simulink model "pmsm_ctrl"  (R2018a)
settings: Solver=FixedStepDiscrete  StartTime=0.0  StopTime=3  FixedStep=FastTsample / 10.  RelTol=1e-3  EnableMultiTasking=on
model workspace (MATLAB code in the model file):
  | cmdLim = Simulink.Parameter;
  | cmdLim.Value = 15;
  | cmdLim.Description = 'Limit for controlling the maximum surface command angle.';
  | cmdLim.Min = 0;
  | cmdLim.Max = 90;
  | cmdLim.DocUnits = 'deg';
  | 
  | dispGain = Simulink.Parameter;
  | dispGain.Value = 0.75;
  | dispGain.Description = 'Gain applied to the displacement error.';
  | dispGain.Min = 0;
  | dispGain.Max = [];
  | dispGain.DocUnits = 'deg/sec/deg';
  | 
  | dispLim = Simulink.Parameter;
  | dispLim.Value = 30;
  | dispLim.Description = 'Limit for controlling the maximum commanded angle.';
  | dispLim.Min = 0;
  | dispLim.Max = 180;
  | dispLim.DocUnits = 'deg';
  | 
  | intGain = Simulink.Parameter;
  | intGain.Value = 0.5;
  | intGain.Description = 'Gain applied to the integral error.';
  | intGain.Min = 0;
  | intGain.Max = [];
  | intGain.DocUnits = 'deg/sec/deg/sec';
  | 
  | intLim = Simulink.Parameter;
  | intLim.Value = 5;
  | intLim.Description = 'Limit for controlling the maximum commanded angle.';
  | intLim.Min = 0;
  | intLim.Max = 90;
  | intLim.DocUnits = 'deg';
  | 
  | rateGain = Simulink.Parameter;
  | rateGain.Value = 2;
  | rateGain.Description = 'Gain applied to the rate error.';
  | rateGain.Min = 0;
  | rateGain.Max = [];
  | rateGain.DocUnits = 'deg/deg/sec';
  | 
  | rateLim = Simulink.Parameter;
  | rateLim.Value = 6;
  | rateLim.Description = 'Limit for controlling the maximum commanded angle.';
  | rateLim.Min = 0;
  | rateLim.Max = 180;
  | rateLim.DocUnits = 'deg/sec';
  | 
  | hdgGain = Simulink.Parameter;
  | hdgGain.Value = 0.015;
undefined symbols (not defined in the file): CalMgrSt_T, Cfg_AnglOfsCalPwmDuty, Cfg_AutoCalEnbl, Cfg_EnblDynComp, Cfg_EnblTrajPlan, Cfg_EncCnts, Cfg_EncOfsCalPwmDuty, Cfg_IfbkCtrlBW, Cfg_IndCalPwmDuty, Cfg_Ls, Cfg_MFlux, Cfg_MtrJm, Cfg_MtrKf, Cfg_MtrKtrq, Cfg_PolePairs, Cfg_ResCalPwmDuty, Cfg_Rs, Cfg_SpdCtrlBW, Cfg_SpdSnsEnbl, Cfg_StepToEncCnts, Cfg_UseObsPosEst, Cfg_VBus, DiscIntNeverNeededParam, DistObs_J, EncCntsToRads, MtrCtrlCal_T, MtrCtrlMd, MtrCtrlMd_T, MtrParams, TsFast, TsMain
libraries: ctrl_lib x13, simulink x10, adrc_lib x2, peTransforms x1
(part 2 of 2)

== system pmsm_ctrl/CtrlFast/Field_Oriented_Controller/ifbk_trq_ctrl/IfbkCtrl/ifbk_q_ctrl ==
  IfbkTgt : Inport
  IfbkAct : Inport  Port=2
  Params : Inport  Port=3
  Bus Selector : BusSelector  OutputSignals=Lest,Rest
  Constant : Constant  Value=Cfg_Ls * Cfg_IfbkCtrlBW
  Constant1 : Constant  Value=Cfg_Rs * Cfg_IfbkCtrlBW
  Constant2 : Constant  Value=Cfg_AutoCalEnbl
  Constant3 : Constant  Value=Cfg_IfbkCtrlBW
  Demux : Demux  Outputs=2
  Mux : Mux  Inputs=2
  Mux1 : Mux  Inputs=2
  PI-Ctrl-Varying-Gains : ctrl_lib/PI-Ctrl-Varying-Gains  ts=TsFast  max_lim=12  min_lim=-12
  Product : Product
  Switch : Switch  Criteria=u2 ~= 0
  Ctrl : Outport
  wires:
  IfbkTgt/1 -> PI-Ctrl-Varying-Gains/1
  IfbkAct/1 -> PI-Ctrl-Varying-Gains/2
  Params/1 -> Bus Selector/1
  Bus Selector/2 -> Mux/2  "<Rest>"
  Bus Selector/1 -> Mux/1  "<Lest>"
  Demux/1 -> PI-Ctrl-Varying-Gains/3
  Demux/2 -> PI-Ctrl-Varying-Gains/4
  Constant/1 -> Mux1/1
  Constant1/1 -> Mux1/2
  Switch/1 -> Demux/1
  Mux/1 -> Product/2
  Constant2/1 -> Switch/2
  Mux1/1 -> Switch/3
  Product/1 -> Switch/1
  Constant3/1 -> Product/1
  PI-Ctrl-Varying-Gains/1 -> Ctrl/1

== system pmsm_ctrl/CtrlFast/Field_Oriented_Controller/ifbk_trq_ctrl/IfbkCtrl/mtr_coupling_bemf_comp ==
  ifbk_q_act : Inport
  mtr_spd_act : Inport  Port=2
  ifbk_d_act : Inport  Port=3
  Enable : EnablePort  StatesWhenEnabling=reset
  Add1 : Sum
  Gain : Gain  Gain=-Cfg_Ls  ParamDataTypeStr=single
      settings: AttributesFormatString=%<Gain>
  Gain2 : Gain  Gain=Cfg_MFlux / Cfg_Ls
      settings: AttributesFormatString=%<Gain>
  Gain3 : Gain  Gain=Cfg_Ls
      settings: AttributesFormatString=%<Gain>
  Gain4 : Gain  Gain=Cfg_PolePairs
      settings: AttributesFormatString=%<Gain>
  Product : Product
  Product1 : Product
  ifbk_q_comp : Outport
  ifbk_d_comp : Outport  Port=2
  wires:
  Gain2/1 -> Add1/2
  Product1/1 -> Add1/1
  ifbk_d_act/1 -> Product1/1
  Product/1 -> Gain/1
  Add1/1 -> Gain3/1
  mtr_spd_act/1 -> Gain4/1
  ifbk_q_act/1 -> Product/2
  Gain3/1 -> ifbk_q_comp/1
  Gain/1 -> ifbk_d_comp/1
  Gain4/1 -> Product/1, Product1/2, Gain2/1

== stateflow chart pmsm_ctrl/CalibRoutines/mtr_ind_ident/IndIdCal ==
  state res_id_init
    en, du:
    CtrlMdRqst = MtrCtrlMd_T.CTRL_MD_RAW_PWM;
    PwmRqst = Cfg_IndCalPwmDuty;
    CalMgrStRqst = CalMgrSt_T.ST_IND_ID;
    CalData_L = -1.0;
  state ind_id_actv
    en:
    ifbk_pos = 0;
    ifbk_neg = 0;
    state pos_cycle
      en, du:
      PwmRqst = Cfg_IndCalPwmDuty;
      ifbk_neg += MtrIfbk;
    state neg_cycle
      en, du:
      PwmRqst = -Cfg_IndCalPwmDuty;
      ifbk_pos += MtrIfbk;
    (default) -> pos_cycle
    pos_cycle -> neg_cycle
    neg_cycle -> pos_cycle
  state done
    en, du:
    CtrlMdRqst = MtrCtrlMd_T.CTRL_MD_OFF;
    CalMgrStRqst = CalMgrSt_T.ST_DONE;
    PwmRqst = 0.;
    di_dt = ((ifbk_pos - ifbk_neg) / (TICK_L_CAL / 2.)) / TsMain;
    CalData_L = Cfg_IndCalPwmDuty * (Cfg_VBus/ 2.) / di_dt;
  (default) -> res_id_init
  res_id_init -> ind_id_actv : [after(TICK_L_CAL_WAIT_SETTLE, tick)] // Wait for current / motor to settle.
  ind_id_actv -> done : [after(TICK_L_CAL, tick)]
  data: CtrlMdRqst output; CalMgrStRqst output; PwmRqst output single; MtrIfbk input; CalData_L data_store_memory; MtrParams parameter; Cfg_IndCalPwmDuty parameter single; TICK_L_CAL_WAIT_SETTLE constant uint32 =30; TICK_L_CAL constant uint32 =1000; ifbk_neg local single =0; ifbk_pos local single =0.; di_dt local single =0.; TsMain parameter; Cfg_VBus parameter single

== stateflow chart pmsm_ctrl/CalibRoutines/mtr_ifbk_ofs_ident/ResIdCal ==
  state mtr_angl_ofs_cal_actv
    en, du:
    CtrlMdRqst = MtrCtrlMd_T.CTRL_MD_RAW_PWM;
    PwmRqst = 0.0;
    CalMgrStRqst = CalMgrSt_T.ST_IFBK_OFS_CAL;
    ifbk_abc_sum = get_mtr_ifbk_sum(MtrIfbk);
    CalData_IfbkOfs_Abc[0] = 0.;
    CalData_IfbkOfs_Abc[1] = 0.;
    CalData_IfbkOfs_Abc[2] = 0.;
  state mtr_ifbk_sum_abc = get_mtr_ifbk_sum(mtr_ifbk_abc) [function]
  state mtr_ifbk_avg_abc = get_mtr_ifbk_avg(mtr_ifbk_sum_abc, ncycles) [function]
  state mtr_angl_ofs_cal_done
    en, du:
    CtrlMdRqst = MtrCtrlMd_T.CTRL_MD_OFF;
    CalMgrStRqst = CalMgrSt_T.ST_DONE;
    PwmRqst = 0.0;
    CalData_IfbkOfs_Abc = get_mtr_ifbk_avg(ifbk_abc_sum, TICK_IFBK_OFS_WAIT_SETTLE);
  (default) -> mtr_angl_ofs_cal_actv
  mtr_angl_ofs_cal_actv -> mtr_angl_ofs_cal_done : [after(TICK_IFBK_OFS_WAIT_SETTLE, tick)] // Wait for motor to settle.
  data: mtr_ifbk_abc function_input size=3; mtr_ifbk_sum_abc function_output; mtr_ifbk_sum_abc function_input size=3; mtr_ifbk_avg_abc function_output; ncycles function_input; CtrlMdRqst output; CalMgrStRqst output; PwmRqst output single; ifbk_abc_sum local single size=3; MtrIfbk input size=3; CalData_IfbkOfs_Abc data_store_memory; TICK_IFBK_OFS_WAIT_SETTLE constant uint32 =500

== stateflow chart pmsm_ctrl/CalibRoutines/enc_ofs_cal_routine/EncOfsCal ==
  state mtr_n_poles_enc_ofs_init
    en:
    TICK_TGT = 8 * Cfg_EncCnts;
    en, du:
    CtrlMdRqst = MtrCtrlMd_T.CTRL_MD_RAW_PWM;
    PwmRqst = Cfg_AnglOfsCalPwmDuty;
    CalMgrStRqst = CalMgrSt_T.ST_ENC_OFS;
    CalData_EncOfs = 0;
    CalData_nPoles = -1;
    Ticks = 0;
    ticks_inc = int32(TICK_TGT / TICK_OFS_CAL_RAMP);
    CalData_EncOfs = EncCnts;
    ticks_start = 0;
    ticks_end = 0;
  state enc_cnts_err
    en, du:
    // When state machine goes into this state, it means that no encoder movement
    // was detected; either because the encoder is not connected, motor has no
    // power or something else. So calibration is finished here.
    // TODO: Signal & handle error.
    ticks_end = 0;
    CalData_nPoles = -1;
    CtrlMdRqst = MtrCtrlMd_T.CTRL_MD_OFF;
    CalMgrStRqst = CalMgrSt_T.ST_FAILED;
    CalData_EncOfs = -Cfg_EncCnts;
  state calc_enc_ofs_move_forward
    en:
    PwmRqst = Cfg_EncOfsCalPwmDuty;
    ticks_start = EncCnts;
    du:
    PwmRqst = Cfg_EncOfsCalPwmDuty;
    Ticks += ticks_inc;
    ticks_end = EncCnts;
  state calc_n_poles
    en, du:
    Ticks = Ticks;
    CalData_nPoles = int32(Ticks / abs(ticks_end - ticks_start))
  state move_back_calc_enc_ofs
    en, du:
    Ticks -= ticks_inc;
  state done
    en, du:
    CtrlMdRqst = MtrCtrlMd_T.CTRL_MD_OFF;
    CalMgrStRqst = CalMgrSt_T.ST_DONE;
    PwmRqst = 0.;
  (default) -> mtr_n_poles_enc_ofs_init
  mtr_n_poles_enc_ofs_init -> calc_enc_ofs_move_forward : [after(TICK_ENC_OFS_WAIT_SETTLE, tick)] // Wait for motor / current to settle.
  calc_enc_ofs_move_forward -> enc_cnts_err [order 1] : [(Ticks >= TICK_TGT) && (abs(ticks_end - ticks_start) < TICK_INC_MIN)]
  calc_enc_ofs_move_forward -> calc_n_poles [order 2] : [(Ticks >= TICK_TGT) ]
  (junction 68) -> enc_cnts_err
  calc_n_poles -> (junction 68) [order 1] : [(CalData_nPoles < POLES_CAL_MIN) || (CalData_nPoles > POLES_CAL_MAX)]
  calc_n_poles -> move_back_calc_enc_ofs [order 2] : [after(1, tick)]
  move_back_calc_enc_ofs -> done : [Ticks <= 0]
  data: Cfg_AnglOfsCalPwmDuty parameter size=1; EncCnts input size=1; CtrlMdRqst output; CalMgrStRqst output; PwmRqst output single; CalData_EncOfs data_store_memory; Ticks output int32; ticks_inc local int32; ticks_tgt local int32; CalData_nPoles data_store_memory; ticks_start local int32; ticks_end local int32; TICK_TGT local int32; TICK_ENC_OFS_WAIT_SETTLE constant uint32 =200; TICK_OFS_CAL_RAMP constant uint32 =500; Cfg_EncCnts parameter; Cfg_EncOfsCalPwmDuty parameter; TICK_INC_MIN constant int32 =100; POLES_CAL_MIN constant int32 =1; POLES_CAL_MAX constant int32 =20
  data TICK_INC_MIN settings: description=During pole calibration, if the encoder does not move at least this number of counts, then it is considered to be faulted (motor did not move), and pole calculation is not possible.
  data POLES_CAL_MIN settings: description=Number of pole pairs minimum limit.
  data POLES_CAL_MAX settings: description=Maximum pole pairs limit.

== stateflow chart pmsm_ctrl/CalibRoutines/mtr_res_ident/ResIdCal ==
  state res_id_init
    en, du:
    CtrlMdRqst = MtrCtrlMd_T.CTRL_MD_RAW_PWM;
    PwmRqst = Cfg_ResCalPwmDuty;
    CalMgrStRqst = CalMgrSt_T.ST_RES_ID;
    ifbk_sum = 0;
    CalData_Res = -1.0;
  state res_id_actv
    en, du:
    ifbk_sum += MtrIfbk;
  state done
    en, du:
    CtrlMdRqst = MtrCtrlMd_T.CTRL_MD_OFF;
    CalMgrStRqst = CalMgrSt_T.ST_DONE;
    PwmRqst = 0.;
    CalData_Res = Cfg_ResCalPwmDuty * (2. / 3.) * (MtrParams.Vdc / 2.) / (ifbk_sum / TICK_R_CAL);
  (default) -> res_id_init
  res_id_init -> res_id_actv : [after(TICK_R_CAL_WAIT_SETTLE, tick)] // Wait for current / motor to settle.
  res_id_actv -> done : [after(TICK_R_CAL, tick)]
  data: CtrlMdRqst output; CalMgrStRqst output; PwmRqst output single; ifbk_sum local single =0.; MtrIfbk input; CalData_Res data_store_memory; MtrParams parameter; Cfg_ResCalPwmDuty parameter single; TICK_R_CAL_WAIT_SETTLE constant uint32 =30; TICK_R_CAL constant uint32 =100
